simulink model "RefModel_RigOutput"  (R2015b)
settings: configuration reference "CenterOutReachConfigSet" (kept outside this file)
undefined symbols (not defined in the file or in its folder): HandSource, macaddr
undefined symbols (not defined in the file): RigInfo
libraries: libBusSerialize x4, simulink x4, xpcnilib x2, slrtlib x1, dspswit3 x1
settings Model: Creator=djoshea  LastModifiedBy=shenoylab
settings ConfigSetRef: SourceLocation=Base Workspace

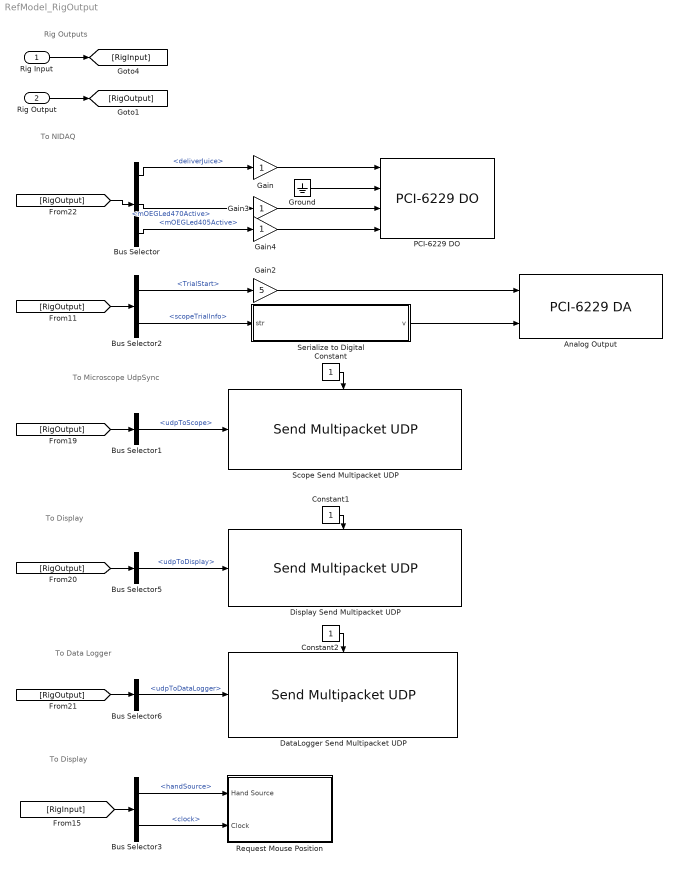
== system RefModel_RigOutput ==
  note: To Display
  note: To NIDAQ
  note: To Microscope UdpSync
  note: To Display
  note: To Data Logger
  note: Rig Outputs
  Rig Input : Inport  OutDataTypeStr=Bus: RigInputBus  PortDimensions=1  Interpolate=off  BusOutputAsStruct=on
  Rig Output : Inport  Port=2  OutDataTypeStr=Bus: RigOutputBus  PortDimensions=1  Interpolate=off  BusOutputAsStruct=on
  Analog Output : xpcnilib/D//A/M Series/PCI-6229 DA  channel=[1 2]  reset=[1]  initValue=[0]  sampletime=0.001  slot=-1
  Bus Selector : BusSelector  OutputSignals=deliverJuice,mOEGLed470Active,mOEGLed405Active
  Bus Selector1 : BusSelector  OutputSignals=udpToScope
  Bus Selector2 : BusSelector  OutputSignals=TrialStart,scopeTrialInfo
  Bus Selector3 : BusSelector  OutputSignals=rigConfig.handSource,clock
  Bus Selector5 : BusSelector  OutputSignals=udpToDisplay
  Bus Selector6 : BusSelector  OutputSignals=udpToDataLogger
  Constant : Constant
  Constant1 : Constant
  Constant2 : Constant
  DataLogger Send Multipacket UDP : libBusSerialize/Send Multipacket UDP  transmitId=8  sourceIP=RigInfo.network.dataLoggerVLAN.sourceIP  sourcePort=RigInfo.network.dataLoggerVLAN.sourcePort  destIP=RigInfo.network.dataLoggerVLAN.broadcastIP  destPort=RigInfo.network.dataLoggerVLAN.destPort  destMac=RigInfo.network.dataLoggerVLAN.broadcastMac  deviceID=RigInfo.network.dataLoggerVLAN.ethernetId  prependHeader=on
  Display Send Multipacket UDP : libBusSerialize/Send Multipacket UDP  transmitId=1  sourceIP=RigInfo.network.displayVLAN.sourceIP  sourcePort=RigInfo.network.displayVLAN.sourcePort  destIP=RigInfo.network.displayVLAN.broadcastIP  destPort=RigInfo.network.displayVLAN.destPort  destMac=RigInfo.network.displayVLAN.broadcastMac  deviceID=RigInfo.network.displayVLAN.ethernetId  prependHeader=on
  Gain : Gain  OutDataTypeStr=double
  Gain2 : Gain  Gain=5  OutDataTypeStr=double
  Gain3 : Gain  OutDataTypeStr=double
  Gain4 : Gain  OutDataTypeStr=double
  Ground : Ground
  PCI-6229 DO : xpcnilib/Digital Output/M Series/PCI-6229 DO  channel=[5 2 3 4]  reset=[1 1 1 1]  initValue=[0 0 0 0]  sampletime=0.001  slot=-1
  Request Mouse Position : Subsystem
  Scope Send Multipacket UDP : libBusSerialize/Send Multipacket UDP  transmitId=1  sourceIP=RigInfo.network.scopeVLAN.sourceIP  sourcePort=RigInfo.network.scopeVLAN.sourcePort  destIP=RigInfo.network.scopeVLAN.broadcastIP  destPort=RigInfo.network.scopeVLAN.destPort  destMac=RigInfo.network.scopeVLAN.broadcastMac  deviceID=RigInfo.network.scopeVLAN.ethernetId  prependHeader=off
  Serialize to Digital : MATLAB Function  TreatAsAtomicUnit=on  mask(Serialize ASCII to Digital Output){bufferSize=RigInfo.outputSizes.trialInfoToScope}
      mask prompts: bufferSize "Buffer Size"
      mask help: Buffers incoming inputs (ASCII strings) and outputs one bit per tick as a trinary signal (0V = low, 2.5 V = pause, 5V = high). Bytes are sent in MSB first order, with a single 2.5V sample sent in between each byte.
  wires:
  Bus Selector3/1 -> Request Mouse Position/1(Hand Source)  "<handSource>"
  [RigOutput] -> Bus Selector2/1
  Bus Selector1/1 -> Scope Send Multipacket UDP/1  "<udpToScope>"
  Bus Selector5/1 -> Display Send Multipacket UDP/1  "<udpToDisplay>"
  Bus Selector6/1 -> DataLogger Send Multipacket UDP/1  "<udpToDataLogger>"
  Constant/1 -> Scope Send Multipacket UDP/Enable
  Constant1/1 -> Display Send Multipacket UDP/Enable
  Constant2/1 -> DataLogger Send Multipacket UDP/Enable
  [RigInput] -> Bus Selector3/1
  [RigOutput] -> Bus Selector1/1
  [RigOutput] -> Bus Selector5/1
  [RigOutput] -> Bus Selector6/1
  [RigOutput] -> Bus Selector/1
  Rig Input/1 -> [RigInput]
  Bus Selector/1 -> Gain/1  "<deliverJuice>"
  Gain/1 -> PCI-6229 DO/1
  Rig Output/1 -> [RigOutput]
  Bus Selector3/2 -> Request Mouse Position/2(Clock)  "<clock>"
  Bus Selector2/1 -> Gain2/1  "<TrialStart>"
  Bus Selector2/2 -> Serialize to Digital/1(str)  "<scopeTrialInfo>"
  Gain2/1 -> Analog Output/1
  Serialize to Digital/1(v) -> Analog Output/2
  Gain3/1 -> PCI-6229 DO/3
  Gain4/1 -> PCI-6229 DO/4
  Bus Selector/2 -> Gain3/1  "<mOEGLed470Active>"
  Bus Selector/3 -> Gain4/1  "<mOEGLed405Active>"
  Ground/1 -> PCI-6229 DO/2

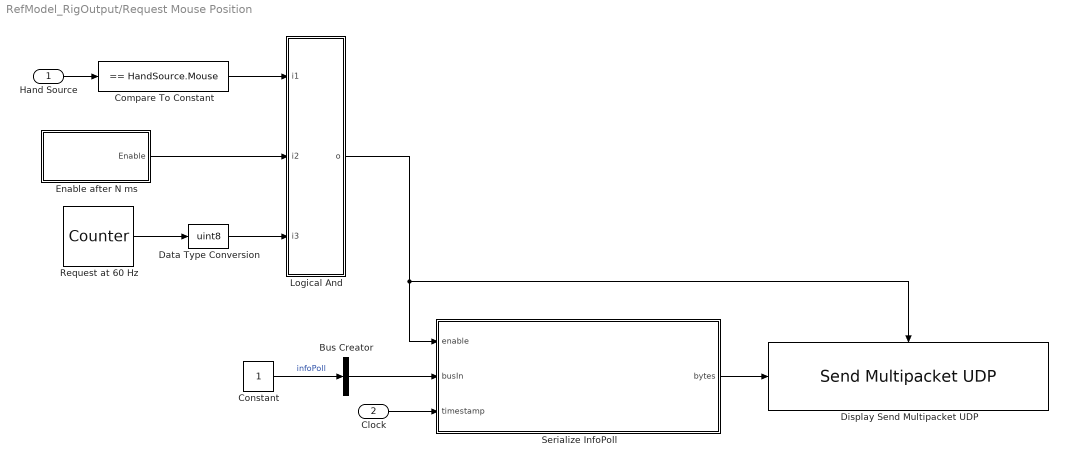
== system RefModel_RigOutput/Request Mouse Position ==
  Hand Source : Inport  OutDataTypeStr=Enum: HandSource  PortDimensions=1
  Clock : Inport  Port=2  OutDataTypeStr=uint32  PortDimensions=1
  Bus Creator : BusCreator  Inputs=1  OutDataTypeStr=Bus: DisplayInfoRequestBus  NonVirtualBus=on
  Compare To Constant : simulink/Logic and Bit Operations/Compare To Constant  relop===  const=HandSource.Mouse  OutDataTypeStr=uint8
  Constant : Constant  OutDataTypeStr=uint8
  Data Type Conversion : DataTypeConversion  OutDataTypeStr=uint8
  Display Send Multipacket UDP : libBusSerialize/Send Multipacket UDP  transmitId=11  sourceIP=RigInfo.network.displayVLAN.sourceIP  sourcePort=RigInfo.network.displayVLAN.sourcePort  destIP=RigInfo.network.displayVLAN.broadcastIP  destPort=RigInfo.network.displayVLAN.destPort  destMac=macaddr('ff:ff:ff:ff:ff:ff')  deviceID=1  prependHeader=on
  Enable after N ms : Subsystem  mask{const=100}
      mask prompts: const "Initial Wait Ticks"
      mask TypeOptions const:
      | Compare
      | To Constant/const
  Logical And : MATLAB Function  TreatAsAtomicUnit=on
  Request at 60 Hz : dspswit3/Counter  Direction=Up  CountEvent=Free running  CounterSize=User defined  MaxCount=16  InitialCount=0  Output=Hit  HitValue=5  ResetInput=off  SamplesPerFrame=1  Ts=0.001  CntDtype=double  HitDtype=Logical
  Serialize InfoPoll : MATLAB Function  AncestorBlock=libBusSerialize/fn2  TreatAsAtomicUnit=on  mask(BusSerialize: serialize block){busType=Bus: DisplayInfoRequestBus, groupType=Parameter, groupName='infoPoll'}
      mask prompts: busType "Bus Type"; groupType "Group Type"; groupName "Group Name"
      mask help: Select the bus type below to serialize.
      mask init:
      | BusSerialize.maskSerializeWithDataLoggerHeaderBlockUpdate(gcb)
  wires:
  Data Type Conversion/1 -> Logical And/3(i3)
  Constant/1 -> Bus Creator/1  "infoPoll"
  Clock/1 -> Serialize InfoPoll/3(timestamp)
  Bus Creator/1 -> Serialize InfoPoll/2(busIn)
  Serialize InfoPoll/1(bytes) -> Display Send Multipacket UDP/1
  Request at 60 Hz/1 -> Data Type Conversion/1
  Logical And/1(o) -> Display Send Multipacket UDP/Enable, Serialize InfoPoll/1(enable)
  Enable after N ms/1(Enable) -> Logical And/2(i2)
  Compare To Constant/1 -> Logical And/1(i1)
  Hand Source/1 -> Compare To Constant/1

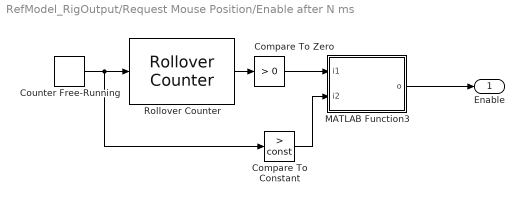
== system RefModel_RigOutput/Request Mouse Position/Enable after N ms ==
  Compare To Constant : simulink/Logic and Bit Operations/Compare To Constant  relop=>  const=const  OutDataTypeStr=uint8
  Compare To Zero : simulink/Logic and Bit Operations/Compare To Zero  relop=>  OutDataTypeStr=uint8
  Counter Free-Running : simulink/Sources/Counter Free-Running  NumBits=16  tsamp=-1
  MATLAB Function3 : MATLAB Function  TreatAsAtomicUnit=on
  Rollover Counter : slrtlib/Incremental Encoder/Utilities/Rollover/Rollover Counter   InitialValue=0  RolloverThreshold=2^15
  Enable : Outport
  wires:
  MATLAB Function3/1(o) -> Enable/1
  Compare To Constant/1 -> MATLAB Function3/2(i2)
  Compare To Zero/1 -> MATLAB Function3/1(i1)
  Rollover Counter/1 -> Compare To Zero/1
  Counter Free-Running/1 -> Compare To Constant/1, Rollover Counter/1

== matlab function RefModel_RigOutput/Serialize to Digital ==
  data: str input uint8; v output double size=1; bufferSize parameter size=1
function v = serializeToDigital(str, bufferSize)
%#codegen
% @djoshea

% serialize in MSB bit first order

OUTPUT_NODATA = 2.5;

persistent pBuffer;
coder.varsize('pBuffer', bufferSize);
if isempty(pBuffer)
    pBuffer = zeros(0, 1, 'uint8');
end

persistent pNextBit;
if isempty(pNextBit)
    pNextBit = 8;
end

persistent pSendSpacer;
if isempty(pSendSpacer)
    pSendSpacer = uint8(0);
end

v = OUTPUT_NODATA;

% append new data to buffer
if ~isempty(str)
    if numel(pBuffer) + numel(str) >= bufferSize
        % flush buffer
        coder.ceval('printf', [char('Warning: overflow on serialize to digital buffer') 10 0]);
        pBuffer = zeros(0, 1, 'uint8');
    end
    
    pBuffer = [pBuffer; str];
end

if pSendSpacer
    % send inter-byte 2.5 v out
    pSendSpacer = uint8(0);

elseif ~isempty(pBuffer)
    % serialize buffer out
    assert(pNextBit <= 8 && pNextBit >= 1);
    bit = bitget(pBuffer(1), pNextBit);
    
    if pNextBit <= 1
        % move to next byte and chop the head off the buffer
        pNextBit = 8;
        if numel(pBuffer) > 1
            pBuffer = pBuffer(2:end);
        else
            pBuffer = zeros(0, 1, 'uint8');
        end
    else    
        % move to next bit (most significant bit first)
        pNextBit = pNextBit - 1;
    end
    
    if bit
        v = 5;
    else
        v = 0;
    end
    
    pSendSpacer = uint8(1);
end

== matlab function RefModel_RigOutput/Request Mouse Position/Enable after N ms/MATLAB Function3 ==
  data: i1 input uint8; o output uint8 size=1; i2 input uint8 size=1
function o = OR(i1, i2)
%#codegen

o = uint8(i1 || i2);

== matlab function RefModel_RigOutput/Request Mouse Position/Logical And ==
  data: i1 input uint8; o output uint8 size=1; i2 input uint8 size=1; i3 input uint8 size=1
function o = AND(i1, i2, i3)
%#codegen

o = uint8(i1 && i2 && i3);

== matlab function RefModel_RigOutput/Request Mouse Position/Serialize InfoPoll ==
  data: enable input uint8 size=1; busIn input Bus: DisplayInfoRequestBus size=1; bytes output uint8 size=45; timestamp input uint32 size=1
function bytes = dataLoggerSerialize(enable, busIn, timestamp)
%#codegen
    if enable
        bytes = serializeBusWithDataLoggerHeader_DisplayInfoRequestBus(busIn, uint8(BusSerialize.GroupTypes.Parameter), uint8('infoPoll'), timestamp);
    else
        bytes = zeros(0, 1, 'uint8');
    end
end
